simulink model "CONTROL_BLOCK"  (R2024b)
settings: configuration reference "MODEL_CONFIG_CHILD" (kept outside this file)
libraries: slpidlib x1
settings Model: Creator=415  LastModifiedBy=415
settings ConfigSetRef: SourceName=MODEL_CONFIG_CHILD  SourceLocation=Base Workspace

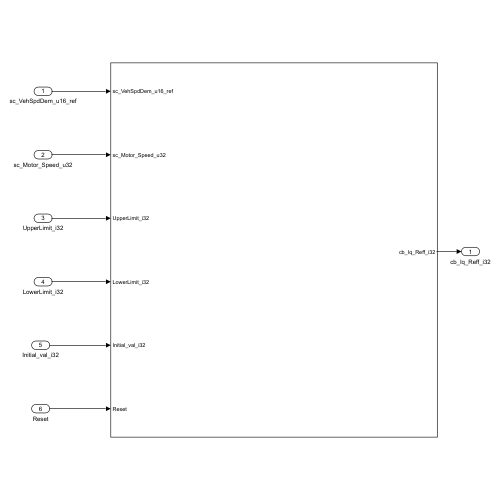
[thumbnail: Simulink's stored preview of the top-level diagram]
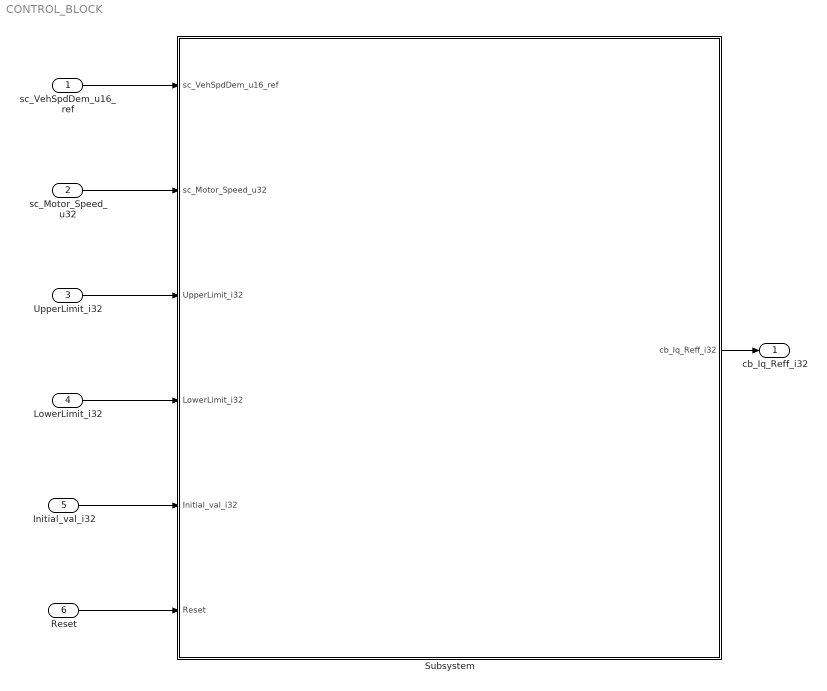
== system CONTROL_BLOCK ==
  sc_VehSpdDem_u16_ref : Inport
  sc_Motor_Speed_u32 : Inport  Port=2
  UpperLimit_i32 : Inport  Port=3
  LowerLimit_i32 : Inport  Port=4
  Initial_val_i32 : Inport  Port=5
  Reset : Inport  Port=6
  Subsystem : Subsystem
  cb_Iq_Reff_i32 : Outport
  wires:
  sc_VehSpdDem_u16_ref/1 -> Subsystem/1(sc_VehSpdDem_u16_ref)
  sc_Motor_Speed_u32/1 -> Subsystem/2(sc_Motor_Speed_u32)
  UpperLimit_i32/1 -> Subsystem/3(UpperLimit_i32)
  LowerLimit_i32/1 -> Subsystem/4(LowerLimit_i32)
  Subsystem/1(cb_Iq_Reff_i32) -> cb_Iq_Reff_i32/1
  Initial_val_i32/1 -> Subsystem/5(Initial_val_i32)
  Reset/1 -> Subsystem/6(Reset)

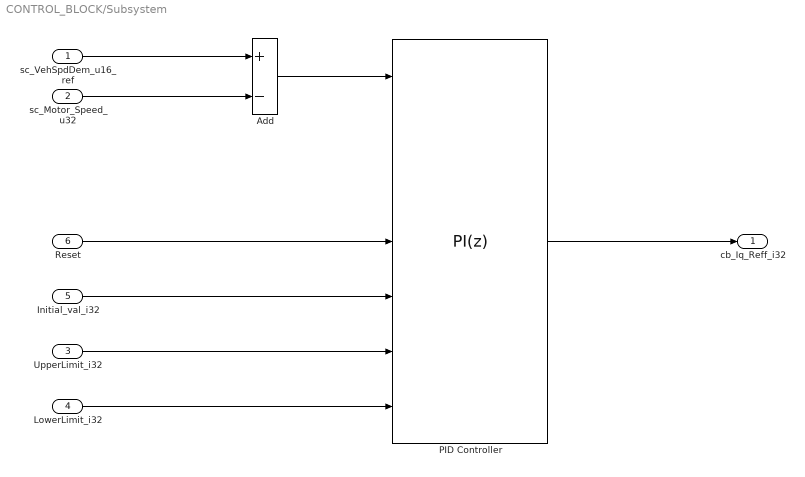
== system CONTROL_BLOCK/Subsystem ==
  sc_VehSpdDem_u16_ref : Inport
  sc_Motor_Speed_u32 : Inport  Port=2
  UpperLimit_i32 : Inport  Port=3
  LowerLimit_i32 : Inport  Port=4
  Initial_val_i32 : Inport  Port=5
  Reset : Inport  Port=6
  Add : Sum  Inputs=+-
  PID Controller : slpidlib/PID Controller  Controller=PI  Form=Parallel  TimeDomain=Discrete-time  UseExternalTs=off  SampleTime=-1  IntegratorMethod=Forward Euler  FilterMethod=Forward Euler  ControllerParametersSource=external  P=1  I=1  UseKiTs=off  D=0  UseExternalDerivativeSource=off  N=100  UseFilter=on  TunerSelectOption=Transfer Function Based (PID Tuner App)  InitialConditionSource=external  InitialConditionForIntegrator=0  InitialConditionForFilter=0  DifferentiatorICPrevScaledInput=0  ExternalReset=rising  TrackingMode=off  Kt=1  LimitOutput=on  SatLimitsSource=external  UpperSaturationLimit=inf  LowerSaturationLimit=-inf  LinearizeAsGain=on  AntiWindupMode=none  Kb=1  LimitIntegrator=off  UpperIntegratorSaturationLimit=inf  LowerIntegratorSaturationLimit=-inf  SaturateOnIntegerOverflow=on  POutMin=[]  POutMax=[]  IOutMin=[]  IOutMax=[]  DOutMin=[]  DOutMax=[]  NOutMin=[]  NOutMax=[]  SumOutMin=[]  SumOutMax=[]  SaturationOutMin=[]  SaturationOutMax=[]  PParamMin=[]  PParamMax=[]  IParamMin=[]  IParamMax=[]  DParamMin=[]  DParamMax=[]  NParamMin=[]  NParamMax=[]  KbParamMin=[]  KbParamMax=[]  KtParamMin=[]  KtParamMax=[]  KbOutMin=[]  KbOutMax=[]  KtOutMin=[]  KtOutMax=[]  IntegratorOutMin=[]  IntegratorOutMax=[]  FilterOutMin=[]  FilterOutMax=[]  SumI1OutMin=[]  SumI1OutMax=[]  SumI2OutMin=[]  SumI2OutMax=[]  SumI3OutMin=[]  SumI3OutMax=[]  SumI4OutMin=[]  SumI4OutMax=[]  SumDOutMin=[]  SumDOutMax=[]  DifferentiatorOutMin=[]  DifferentiatorOutMax=[]  FilterDiffOutCoefMin=[]  FilterDiffOutCoefMax=[]  ReciprocalOutMin=[]  ReciprocalOutMax=[]  SumDenOutMin=[]  SumDenOutMax=[]  SumNumOutMin=[]  SumNumOutMax=[]  DivideOutMin=[]  DivideOutMax=[]  UdiffTsProdOutMin=[]  UdiffTsProdOutMax=[]  NTsProdOutMin=[]  NTsProdOutMax=[]  UintegralTsProdOutMin=[]  UintegralTsProdOutMax=[]  UngainTsProdOutMin=[]  UngainTsProdOutMax=[]  ClampingZeroOutDataTypeStr=Inherit: Inherit via back propagation  ClampingZeroOutMin=[]  ClampingZeroOutMax=[]  FilterDenConstantOutDataTypeStr=Inherit: Inherit via back propagation  FilterDenConstantOutMin=[]  FilterDenConstantOutMax=[]  PCopyOutDataTypeStr=Inherit: Inherit via back propagation  PCopyOutMin=[]  PCopyOutMax=[]  NCopyOutDataTypeStr=Inherit: Inherit via back propagation  NCopyOutMin=[]  NCopyOutMax=[]  IntegratorContinuousStateAttributes=''  IntegratorStateMustResolveToSignalObject=off  IntegratorRTWStateStorageClass=Auto  FilterContinuousStateAttributes=''  FilterStateMustResolveToSignalObject=off  FilterRTWStateStorageClass=Auto  ParallelPVariant=ExternalParameters  IdealPVariant=Disabled  IVariant=ExternalParameters  DVariant=Disabled  IntegratorVariant=Discrete  SatVariant=External  AWVariant=Passthrough  PCopyVariant=Disabled  TRVariant=Disabled  FdbkBlocksVariant=Forward  IdealPFdbkVariant=Disabled  SatFdbkVariant=Disabled  DerivativeFilterVariant=Disabled  NVariant=Disabled  NCopyVariant=Disabled_SignalSpec  FilterICVariant=Disabled  IntegratorICVariant=ExternalICs  ExternalResetVariant=ExternalReset  TRSumVariant=Passthrough  SumFdbkVariant=Disabled  SumVariant=Sum_PI  TsampFilterVariant=InternalTs  TsampNgainVariant=Passthrough  TsampIntegralVariant=Disabled_SignalSpec  ExternalSaturationOutDataTypeStr=Inherit: Same as second input  DerivativeSourceVariant=Disabled  PreIntVariant=InternalPreInt
  cb_Iq_Reff_i32 : Outport
  wires:
  Add/1 -> PID Controller/1
  sc_VehSpdDem_u16_ref/1 -> Add/1
  sc_Motor_Speed_u32/1 -> Add/2
  UpperLimit_i32/1 -> PID Controller/6
  LowerLimit_i32/1 -> PID Controller/7
  PID Controller/1 -> cb_Iq_Reff_i32/1
  Initial_val_i32/1 -> PID Controller/5
  Reset/1 -> PID Controller/4
